simulink model "Ex_1_2_cl"  (R2020a)
settings: Solver=VariableStepAuto  StartTime=0.0  StopTime=10.0  RelTol=1e-3
settings Model: Creator=dimit  LastModifiedBy=dimit

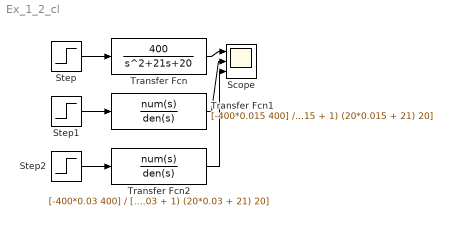
== system Ex_1_2_cl ==
  Scope : Scope  NumInputPorts=3
  Step : Step  Time=0  SampleTime=0
  Step1 : Step  Time=0  SampleTime=0
  Step2 : Step  Time=0  SampleTime=0
  Transfer Fcn : TransferFcn  Numerator=[400]  Denominator=[0 1 21 20]
  Transfer Fcn1 : TransferFcn  Numerator=[-400*0.015 400]  Denominator=[0.015 (21*0.015 + 1) (20*0.015 + 21) 20]
  Transfer Fcn2 : TransferFcn  Numerator=[-400*0.03 400]  Denominator=[0.015 (21*0.03 + 1) (20*0.03 + 21) 20]
  wires:
  Step2/1 -> Transfer Fcn2/1
  Step1/1 -> Transfer Fcn1/1
  Transfer Fcn1/1 -> Scope/2
  Transfer Fcn2/1 -> Scope/3
  Step/1 -> Transfer Fcn/1
  Transfer Fcn/1 -> Scope/1
